simulink model "pitch_x_test"  (R2020a)
settings: Solver=VariableStepAuto  StartTime=0.0  StopTime=30  RelTol=1e-3
values from neighbouring files (symbols this model uses):
  D_pi = 0.002    [test.m]
  D_x = -0.1    [test.m]
  g = 9.8    [test.m]
  I_pi = 0.01    [test.m]
  Iyy = 0.0000716914    (= 7.16914e-05)    [test.m]
  P_pi = 0.013    [test.m]
  P_x = -0.24    [test.m]
settings Model: Creator=denjo  LastModifiedBy=denjo

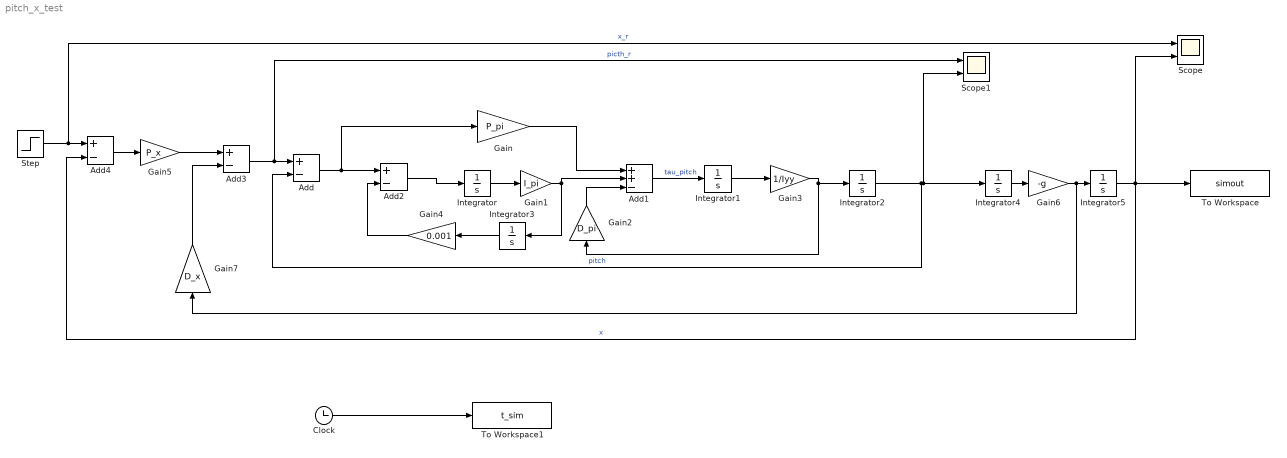
== system pitch_x_test ==
  Add{,2..4} (4 alike) : Sum  Inputs=+-
  Add1 : Sum  Inputs=++-
  Clock : Clock
  Gain : Gain  Gain=P_pi
  Gain1 : Gain  Gain=I_pi
  Gain2 : Gain  Gain=D_pi
  Gain3 : Gain  Gain=1/Iyy
  Gain4 : Gain  Gain=0.001
  Gain5 : Gain  Gain=P_x
  Gain6 : Gain  Gain=-g
  Gain7 : Gain  Gain=D_x
  Integrator{,1..5} (6 alike) : Integrator
  Scope : Scope  NumInputPorts=2
  Scope1 : Scope  NumInputPorts=2
  Step : Step  Time=5  After=10  SampleTime=0
  To Workspace : ToWorkspace  VariableName=simout  SampleTime=-1
  To Workspace1 : ToWorkspace  VariableName=t_sim  SampleTime=-1
  wires:
  Integrator/1 -> Gain1/1
  Add/1 -> Add2/1, Gain/1
  Gain/1 -> Add1/1
  Gain1/1 -> Add1/2, Integrator3/1
  Add1/1 -> Integrator1/1  "tau_pitch"
  Integrator1/1 -> Gain3/1
  Gain3/1 -> Gain2/1, Integrator2/1
  Clock/1 -> To Workspace1/1
  Integrator3/1 -> Gain4/1
  Add2/1 -> Integrator/1
  Gain6/1 -> Gain7/1, Integrator5/1
  Integrator2/1 -> Integrator4/1, Scope1/2, Add/2  "pitch"
  Integrator4/1 -> Gain6/1
  Add3/1 -> Scope1/1, Add/1  "picth_r"
  Gain5/1 -> Add3/1
  Step/1 -> Scope/1, Add4/1  "x_r"
  Add4/1 -> Gain5/1
  Integrator5/1 -> Scope/2, To Workspace/1, Add4/2  "x"
  Gain4/1 -> Add2/2
  Gain7/1 -> Add3/2
  Gain2/1 -> Add1/3
